simulink model "lab10_1"  (R2016a)
settings: Solver=ode45  StartTime=0  StopTime=10.0  MaxStep=0.1  RelTol=1e-3
settings Model: Creator=Student  LastModifiedBy=Student

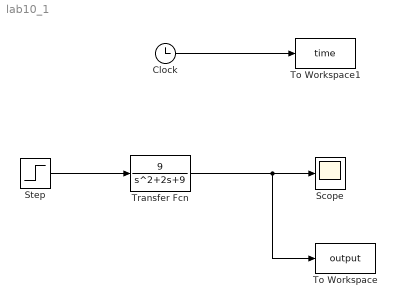
== system lab10_1 ==
  Clock : Clock
  Scope : Scope
  Step : Step  SampleTime=0
  To Workspace : ToWorkspace  VariableName=output  SampleTime=-1
  To Workspace1 : ToWorkspace  VariableName=time  SampleTime=-1
  Transfer Fcn : TransferFcn  Numerator=[9]  Denominator=[1 2 9]
  wires:
  Clock/1 -> To Workspace1/1
  Step/1 -> Transfer Fcn/1
  Transfer Fcn/1 -> To Workspace/1, Scope/1
